simulink model "ask"  (R2020a)
settings: Solver=VariableStepAuto  StartTime=0.0  StopTime=10  RelTol=1e-3
undefined symbols (not defined in the file or in its folder): fdesignblkfcn, gcbh
libraries: commchan3 x1, simulink x1, dspfdesign x1, commseqgen3 x1
settings Model: Creator=Владимир  LastModifiedBy=uzend
settings DataIOCC: ReturnWorkspaceOutputs=off
settings DebuggingCC: ArithmeticOperatorsInVariantConditions=warning
settings SFSimCC: SimUseLocalCustomCode=off  CustomCodeUndefinedFunction=UseInterfaceOnly
settings RTWCC: RTWUseLocalCustomCode=off

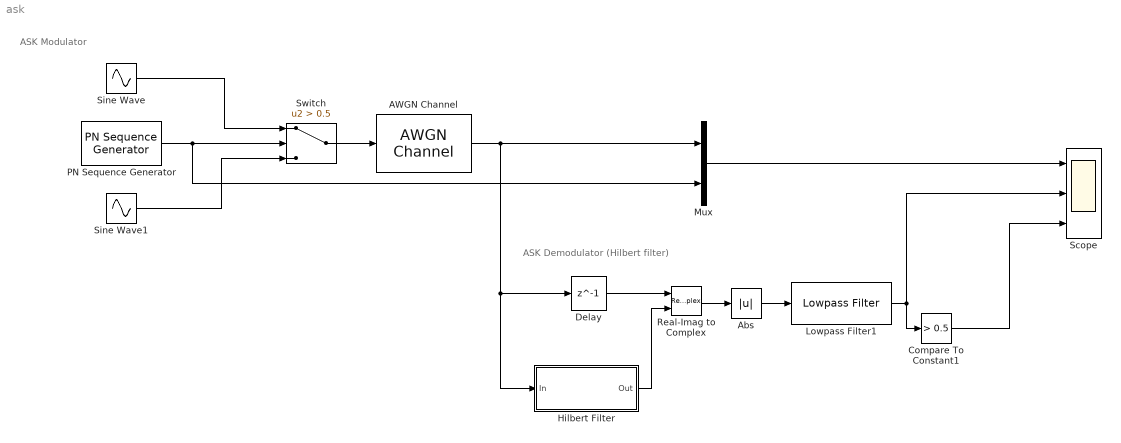
== system ask ==
  note: ASK Demodulator (Hilbert filter)
  note: ASK Modulator
  AWGN Channel : commchan3/AWGN Channel  InputProcessing=Columns as channels (frame based)  seed=67  noiseMode="Signal to noise ratio  (SNR)"  EbNodB=40  EsNodB=10  SNRdB=25  bitsPerSym=1  Ps=1  Tsym=1  variance=1
  Abs : Abs
  Compare To Constant1 : simulink/Logic and Bit Operations/Compare To Constant  relop=>  const=0.5  OutDataTypeStr=boolean
  Delay : Delay  DelayLength=1  InitialCondition=0
  Hilbert Filter : Subsystem  DialogController=fdesignblkfcn  InitFcn=fdesignblkfcn(gcbh, {'InitFcn'});  mask(Hilbert Filter){}
      mask help: Design a Hilbert filter
      settings: CopyFcn=fdesignblkfcn(gcbh, {'CopyFcn'});
      mask Help: helpview(mapfilelocation('dsp'), 'dsphilbertfilter');
      mask Display: disp('Hilbert')
  Lowpass Filter1 : dspfdesign/Lowpass Filter  FilterType=FIR  DesignForMinimumOrder=on  FilterOrder=50  PassbandFrequency=2  StopbandFrequency=4  PassbandRipple=1  StopbandAttenuation=60  InheritSampleRate=on  SampleRate=1000  SimulateUsing=Interpreted execution  roundingMode=Floor  coeffsDataTypeStr=fixdt(1,16)
  Mux : Mux  Inputs=2
  PN Sequence Generator : commseqgen3/PN Sequence Generator  poly='z^6 + z + 1'  ini_sta=[0 0 0 1 0 1]  outBitMaskSource=Dialog parameter  shift=0  outVarSiz=off  maxOutSizeMode=Dialog parameter  maxOutSize=[10 1]  Ts=1  sampPerFrame=1  reset=off  bitPackedOutputs=off  outDataType=double  numPackedBits=8  bitPackDataSigned=off  bitPackedOutDType=double
  Real-Imag to Complex : RealImagToComplex
  Scope : Scope  NumInputPorts=3
  Sine Wave : Sin  Frequency=2*pi*10  SampleTime=0.001
  Sine Wave1 : Sin  Amplitude=0.1  Frequency=2*pi*10  SampleTime=0.001
  Switch : Switch  Criteria=u2 > Threshold  Threshold=0.5
  wires:
  PN Sequence Generator/1 -> Mux/2, Switch/2
  Switch/1 -> AWGN Channel/1
  Mux/1 -> Scope/1
  Sine Wave/1 -> Switch/1
  Sine Wave1/1 -> Switch/3
  AWGN Channel/1 -> Mux/1, Delay/1, Hilbert Filter/1(In)
  Lowpass Filter1/1 -> Scope/2, Compare To Constant1/1
  Delay/1 -> Real-Imag to Complex/1
  Hilbert Filter/1(Out) -> Real-Imag to Complex/2
  Real-Imag to Complex/1 -> Abs/1
  Abs/1 -> Lowpass Filter1/1
  Compare To Constant1/1 -> Scope/3

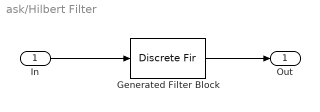
== system ask/Hilbert Filter ==
  In : Inport
  Generated Filter Block : DiscreteFir  Tag=BlockMethodSubSystem  Coefficients=[-0.026449858259791379 -0.00578355491829027 -0.016572261903348456 -0.0095390561131982743 -0.022461390535071568 -0.014999256435125952 -0.030323967074738556 -0.023012528163449009 -0.041429315821655127 -0.035762828939278346 -0.05911752381753177 -0.059034685410808696 -0.094459906652176406 -0.11739830204172252 -0.21797718993610349 -0.62869353747279177 0.62869353747279177 0.21797718993610349 0.11739830204172252 0.094459906652176406 0.059034685410808696 0.05911752381753177 0.035762828939278346 0.041429315821655127 0.023012528163449009 0.030323967074738556 0.014999256435125952 0.022461390535071568 0.0095390561131982743 0.016572261903348456 0.00578355491829027 0.026449858259791379]  InputProcessing=Columns as channels (frame based)
  Out : Outport  VectorParamsAs1DForOutWhenUnconnected=off
  wires:
  Generated Filter Block/1 -> Out/1
  In/1 -> Generated Filter Block/1
